simulink model "spwm"  (R2024a)
settings: Solver=ode45  StartTime=0.0  StopTime=0.03  RelTol=1e-3  EnableMultiTasking=on
libraries: spsMosfetLib x6, spsDCVoltageSourceLib x1, spsSawtoothGeneratorLib x1, spsThreePhaseSeriesRLCLoadLib x1, spsThreePhaseVIMeasurementLib x1, sps_lib x1
settings Model: Creator=Student  LastModifiedBy=harik
settings SolverCC: AlgebraicLoopSolver=TrustRegion
settings DataIOCC: LimitDataPoints=on  SaveFormat=Array  ReturnWorkspaceOutputs=off
settings OptimizationCC: LifeSpan=inf
settings DebuggingCC: UnderspecifiedInitializationDetection=Classic  MergeDetectMultiDrivingBlocksExec=none  SolverPrmCheckMsg=warning  UnconnectedInputMsg=warning  UnconnectedOutputMsg=warning  UnconnectedLineMsg=warning  SFUnexpectedBacktrackingDiag=warning  SFNoUnconditionalDefaultTransitionDiag=warning  SFExecutionAtInitializationDiag=none  ArithmeticOperatorsInVariantConditions=warning
settings HardwareCC: ProdBitPerPointer=32  ProdBitPerSizeT=32  ProdBitPerPtrDiffT=32  ProdLargestAtomicFloat=None  ProdIntDivRoundTo=Undefined  ProdEndianess=Unspecified  ProdWordSize=32  ProdHWDeviceType=32-bit Generic
settings ModelReferenceCC: PropagateSignalLabelsOutOfModel=off
settings SFSimCC: SimUseLocalCustomCode=off  CustomCodeUndefinedFunction=UseInterfaceOnly
settings RTWCC: RTWUseLocalCustomCode=off  GPUComputeCapability=3.5
settings CodeAppCC: StateflowObjectComments=on
settings GRTTargetCC: TargetLangStandard=C89/C90 (ANSI)
settings ConfigComp: CovMetricSettings=dw  CovSaveCumulativeToWorkspaceVar=on  CovSaveSingleToWorkspaceVar=on  CovExternalEMLEnable=off
settings SimscapeCC: SimscapeNormalizeSystem=off

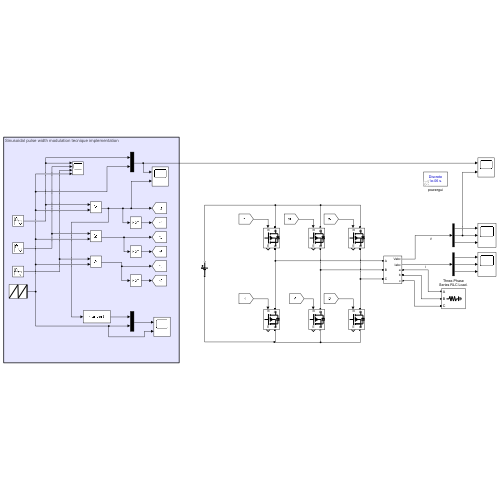
[thumbnail: Simulink's stored preview of the top-level diagram]
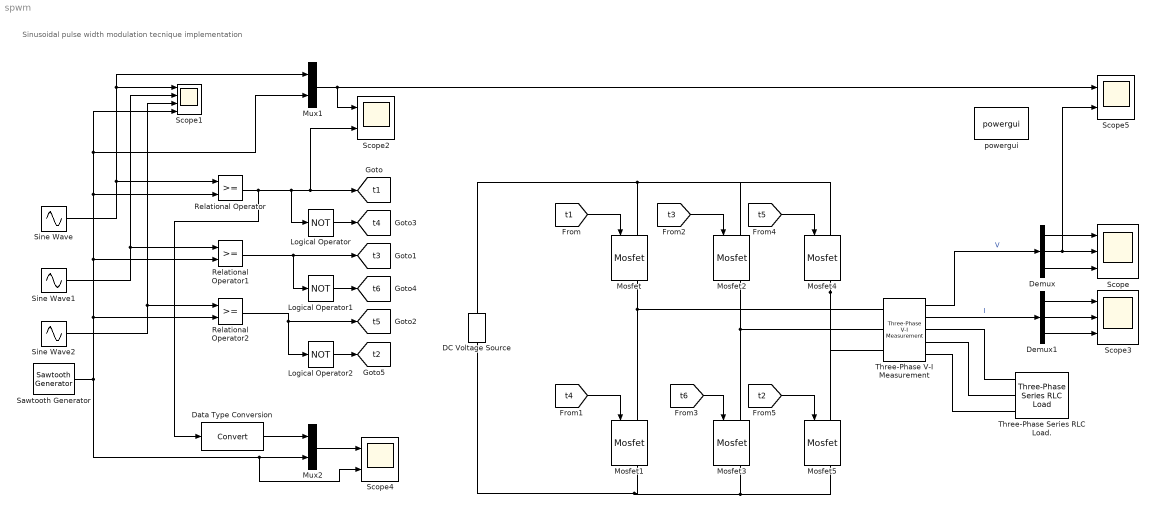
== system spwm ==
  note: Sinusoidal pulse width modulation tecnique implementation
  DC Voltage Source : spsDCVoltageSourceLib/DC Voltage Source  Amplitude=100  Measurements=Voltage
  Data Type Conversion : DataTypeConversion  SaturateOnIntegerOverflow=off  RndMeth=Floor
  Demux : Demux  Outputs=3
  Demux1 : Demux  Outputs=3
  Logical Operator : Logic  Operator=NOT  AllPortsSameDT=off  OutDataTypeStr=boolean
  Logical Operator1 : Logic  Operator=NOT  AllPortsSameDT=off  OutDataTypeStr=boolean
  Logical Operator2 : Logic  Operator=NOT  AllPortsSameDT=off  OutDataTypeStr=boolean
  Mosfet{,1..5} (6 alike) : spsMosfetLib/Mosfet  Ron=0.1  Lon=0  Rd=0.01  Vfd=0  IC=0  Rs=1e5  Cs=inf  Measurements=on
  Mux1 : Mux  Inputs=2
  Mux2 : Mux  Inputs=2
  Relational Operator : RelationalOperator  OutDataTypeStr=boolean  InputSameDT=off
  Relational Operator1 : RelationalOperator  OutDataTypeStr=boolean  InputSameDT=off
  Relational Operator2 : RelationalOperator  OutDataTypeStr=boolean  InputSameDT=off
  Sawtooth Generator : spsSawtoothGeneratorLib/Sawtooth Generator  Freq=1e3  Phase=0  Ts=1/1000000
  Scope : Scope  NumInputPorts=3
  Scope1 : Scope  NumInputPorts=4
  Scope2 : Scope  NumInputPorts=2
  Scope3 : Scope  NumInputPorts=3
  Scope4 : Scope  NumInputPorts=2
  Scope5 : Scope  NumInputPorts=2
  Sine Wave : Sin  Frequency=2*pi*50  SampleTime=1/10000
  Sine Wave1 : Sin  Frequency=2*pi*50  Phase=2*pi/3  SampleTime=1/10000
  Sine Wave2 : Sin  Frequency=2*pi*50  Phase=-2*pi/3  SampleTime=1/10000
  Three-Phase Series RLC Load. : spsThreePhaseSeriesRLCLoadLib/Three-Phase Series RLC Load  LConnTagsString=A|B|C  Configuration=Y (grounded)  NominalVoltage=1000  Vabc=[1e3 1e3 1e3]  Vabcp=[1e3 1e3 1e3]  NominalFrequency=50  UnbalancedPower=off  ActivePower=10e3  InductivePower=0  CapacitivePower=0  Pabc=[10e3 9e3 11e3]  QLabc=[100 90 110]  QCabc=[100 90 110]  Pabcp=[10e3 9e3 11e3]  QLabcp=[100 90 110]  QCabcp=[100 90 110]  Measurements=None  LoadType=constant Z
  Three-Phase V-I Measurement : spsThreePhaseVIMeasurementLib/Three-Phase V-I Measurement  VoltageMeasurement=phase-to-phase  SetLabelV=off  LabelV=Vabc  Vpu=off  VpuLL=off  CurrentMeasurement=yes  SetLabelI=off  LabelI=Iabc  Ipu=off  Pbase=100e6  Vbase=500e3  OutputType=Complex  PhasorSimulation=off  PSBequivalent=0
  powergui : sps_lib/powergui  Priority=1  SimulationMode=Discrete  SampleTime=1e-6  frequency=60  Iterations=50  frequencyindice=0  Pbase=100e6  ErrMax=1e-4  UnitsV=kV  UnitsW=MW  buscounter=0  FunctionMessages=off  echomessages=off  EnableUseOfTLC=off  CurrentSourceSwitches=off  DisableSnubberDevices=off  DisableRonSwitches=off  DisableVfSwitches=off  DisplayEquations=off  AutomaticDiscreteSolvers=off  SolverType=Tustin  Interpol=off  ExternalGateDelay=off  methode=off  Ts=0  x0status=blocks  SPID=off  SwTol=0  HookPort=off  NonlinearTolerance=1e-4  nMaxIteration=100  ContinueOnMaxIteration=off  RestoreLinks=warning  ResistiveCurrentMeasurement=off  Frange=[0:2:500]  Ylog=off  Xlog=on  ShowGrid=off  save=off  variable=ZData  structure=vab  ZoomFFT=off  StartTime=0.0  cycles=3  DisplayStyle=1  fundamental=50  FreqAxis=off  MaxFrequency=1000  frequencyindicesteady=1  RmsSteady=1  display=off
  tag scope: t1=global, t2=global, t3=global, t4=global, t5=global, t6=global
  wires:
  [t1] -> Mosfet/1
  [t3] -> Mosfet2/1
  [t4] -> Mosfet1/1
  [t6] -> Mosfet3/1
  [t2] -> Mosfet5/1
  [t5] -> Mosfet4/1
  Three-Phase V-I Measurement/1 -> Demux/1  "V"
  Demux/1 -> Scope/1
  Demux/2 -> Scope5/2, Scope/2
  Demux/3 -> Scope/3
  Three-Phase V-I Measurement/2 -> Demux1/1  "I"
  Relational Operator2/1 -> Logical Operator2/1, [t5]
  Logical Operator2/1 -> [t2]
  Logical Operator1/1 -> [t6]
  Logical Operator/1 -> [t4]
  Mux1/1 -> Scope2/1, Scope5/1
  Sine Wave1/1 -> Relational Operator1/1, Scope1/2
  Relational Operator1/1 -> Logical Operator1/1, [t3]
  Sine Wave2/1 -> Scope1/3, Relational Operator2/1
  Sine Wave/1 -> Mux1/1, Scope1/1, Relational Operator/1
  Mux2/1 -> Scope4/1
  Sawtooth Generator/1 -> Scope4/2, Mux2/2, Scope1/4, Mux1/2, Relational Operator/2, Relational Operator1/2, Relational Operator2/2
  Relational Operator/1 -> Data Type Conversion/1, Logical Operator/1, Scope2/2, [t1]
  Data Type Conversion/1 -> Mux2/1
  Demux1/1 -> Scope3/1
  Demux1/2 -> Scope3/2
  Demux1/3 -> Scope3/3
  connections:
  DC Voltage Source/LConn1 -- Mosfet1/RConn1 -- Mosfet5/RConn1 -- Mosfet3/RConn1
  Mosfet/LConn1 -- Mosfet2/LConn1 -- Mosfet4/LConn1 -- DC Voltage Source/RConn1
  Mosfet/RConn1 -- Three-Phase V-I Measurement/LConn1 -- Mosfet1/LConn1
  Mosfet2/RConn1 -- Three-Phase V-I Measurement/LConn2 -- Mosfet3/LConn1
  Mosfet4/RConn1 -- Mosfet5/LConn1 -- Three-Phase V-I Measurement/LConn3
  Three-Phase V-I Measurement/RConn2 -- Three-Phase Series RLC Load./LConn2
  Three-Phase V-I Measurement/RConn1 -- Three-Phase Series RLC Load./LConn1
  Three-Phase V-I Measurement/RConn3 -- Three-Phase Series RLC Load./LConn3
